simulink model "test_OSF"  (R2020b)
settings: Solver=VariableStepAuto  StartTime=0.0  StopTime=10  RelTol=1e-3
undefined symbols (not defined in the file): A, B, C, D, G, K_SF
settings Model: Creator=10911  LastModifiedBy=10911

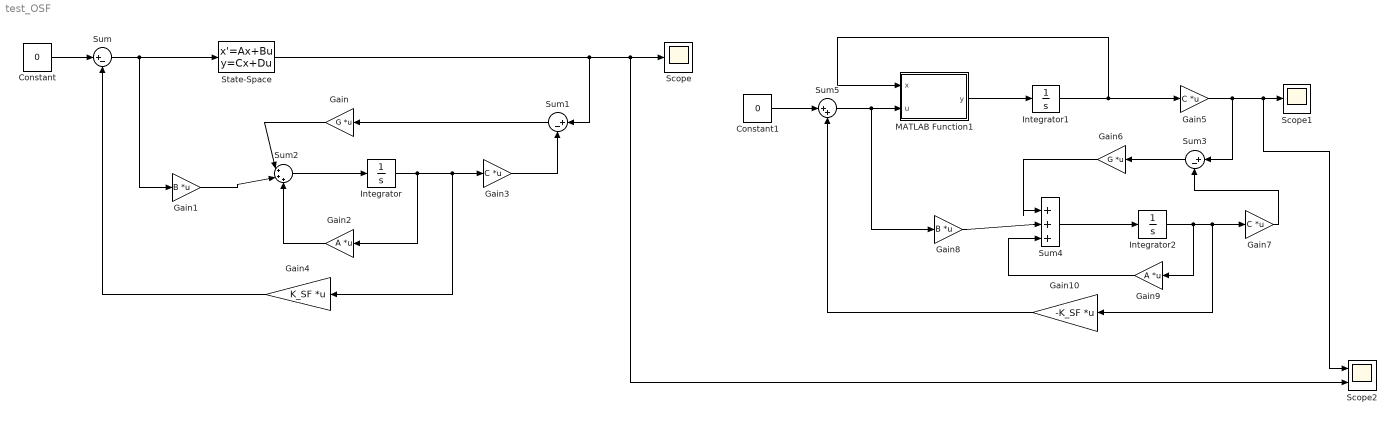
== system test_OSF ==
  Constant : Constant  Value=0
  Constant1 : Constant  Value=0
  Gain : Gain  Gain=G  Multiplication=Matrix(K*u)
  Gain1 : Gain  Gain=B  Multiplication=Matrix(K*u)
  Gain10 : Gain  Gain=-K_SF  Multiplication=Matrix(K*u)
  Gain2 : Gain  Gain=A  Multiplication=Matrix(K*u)
  Gain3 : Gain  Gain=C  Multiplication=Matrix(K*u)
  Gain4 : Gain  Gain=K_SF  Multiplication=Matrix(K*u)
  Gain5 : Gain  Gain=C  Multiplication=Matrix(K*u)
  Gain6 : Gain  Gain=G  Multiplication=Matrix(K*u)
  Gain7 : Gain  Gain=C  Multiplication=Matrix(K*u)
  Gain8 : Gain  Gain=B  Multiplication=Matrix(K*u)
  Gain9 : Gain  Gain=A  Multiplication=Matrix(K*u)
  Integrator : Integrator  InitialCondition=[0;0;0.1;0]
  Integrator1 : Integrator  InitialCondition=[0 0 0.1 0]
  Integrator2 : Integrator  InitialCondition=[0 0 0.1 0]
  MATLAB Function1 : MATLAB Function  TreatAsAtomicUnit=on
  Scope : Scope
  Scope1 : Scope
  Scope2 : Scope  NumInputPorts=2
  State-Space : StateSpace  A=A  B=B  C=C  D=D  InitialCondition=[0;0;0.1;0]
  Sum : Sum  Inputs=|+-
  Sum1 : Sum  Inputs=|+-
  Sum2 : Sum  Inputs=|+++
  Sum3 : Sum  Inputs=|+-
  Sum4 : Sum  Inputs=|+++
  Sum5 : Sum  Inputs=|++
  wires:
  Gain1/1 -> Sum2/2
  Gain4/1 -> Sum/2
  Sum1/1 -> Gain/1
  Sum/1 -> Gain1/1, State-Space/1
  Integrator/1 -> Gain4/1, Gain3/1, Gain2/1
  Gain/1 -> Sum2/1
  Gain2/1 -> Sum2/3
  Gain3/1 -> Sum1/2
  Sum2/1 -> Integrator/1
  State-Space/1 -> Sum1/1, Scope2/2, Scope/1
  Constant/1 -> Sum/1
  Gain6/1 -> Sum4/1
  Sum4/1 -> Integrator2/1
  Integrator1/1 -> MATLAB Function1/1(x), Gain5/1
  Sum3/1 -> Gain6/1
  Gain9/1 -> Sum4/3
  Gain5/1 -> Sum3/1, Scope2/1, Scope1/1
  Gain8/1 -> Sum4/2
  Gain7/1 -> Sum3/2
  Integrator2/1 -> Gain10/1, Gain7/1, Gain9/1
  MATLAB Function1/1(y) -> Integrator1/1
  Constant1/1 -> Sum5/1
  Sum5/1 -> Gain8/1, MATLAB Function1/2(u)
  Gain10/1 -> Sum5/2

== matlab function test_OSF/MATLAB Function1 ==
  data: x input; y output; u input
function y = fcn(x,u)
M = 1;
m = 0.1;
l = 0.5;
g = 9.8;
x1=x(1);
x2=x(2);
x3=x(3);
x4=x(4);

dx1 = x2;
dx2 =(u + m*l*x4*x4*sin(x3) - m*g*sin(x3)*cos(x3))/(M + m - m*cos(x3)*cos(x3));
dx3 = x4;
dx4 =(-u*cos(x3) + (M+m)*g*sin(x3) - m*l*x4*x4*sin(x3)*cos(x3))/((M+m)*l - m*l*cos(x3)*cos(x3));
y = [dx1;dx2;dx3;dx4];
